simulink model "Modele_MS_V1"  (R2019b)
settings: Solver=ode23t  StartTime=0.0  StopTime=3  MaxStep=1e-3  RelTol=1e-3  EnableMultiTasking=on
InitFcn:
  | % Modelisation de la Machine Synchrone
  | 
  | % Constantes
  | 
  | Rs = 0.001;
  | Rdd = 0.01 ;
  | Rdq = Rdd ;
  | Rf = 7 ;
  | Ld = 1.59e-2 ;
  | Lq = Ld ;
  | Lf = 7 ;
  | Ldd = 7e-4 ;
  | Ldq = Ldd ;
  | Maf = 0.259 ;
  | Madd = 2.5e-3 ;
  | Madq = Madd ;
  | Mfdd = 6.8e-2 ;
  | npp = 2 ;
  | J = 0.1 ;
  | 
  | w = 2*pi*50 ;
  | 
  | Omega = w/npp ;
  | 
  | 
  | % Matrices
  | 
  | % V = [Vd Vq 0 0 Vf] ;
  | 
  | % I = [Id Iq Idd Idq If] ;
  | 
  | % F = [Fd Fq Fdd Fdq Ff] ;
  | 
  | L = [ Ld			0		Madd		0			Maf ;
  |       0			Lq		0			Madq		0 			;
  |       1.5*Madd	0		Ldd		0			Mfdd ;
  |       0        1.5*Madq			0			Ldq	0 ;
  |       1.5*Maf	0		Mfdd		0			Lf ] ;
  | 
  | L1 = inv(L) ;
  | 
  | R = [ Rs 0  0   0   0 ;
  |       0  Rs 0   0   0 ;
  |       0  0  Rdd 0   0 ;
  |       0  0  0   Rdq 0 ;
  |       0  0  0   0   Rf ] ;
  | 
  | D = [ 0 -1 0 0 0 ;
  |        1  0 0 0 0 ;
  |        0  0 0 0 0 ;
  |        0  0 0 0 0 ;
  |        0  0 0 0 0 ] ;
  | 
  |     Cl = (1/3)*[ 2  -1      -1 ;
  |      	  	        0  sqrt(3) -sqrt(3) ;
  |                   1  1       1 ] ;
  | 
  |      Cl1 = inv(Cl);
  | 
  | 
  | 
  | Clark=2/3*[	1		-1/2		-1/2
  | 	        0		sqrt(3)/2	-sqrt(3)/2
  | 	        1/2		1/2		1/2		]
  | 
  | InvClark=inv(Clark)
  | 
  | LVIDE=[Ldd   Mfdd
  |         Mfdd    Lf];
  | L2=inv(LVIDE);
  | RVIDE=[Rdd   0
  |         0    Rf];
undefined symbols (not defined in the file or in its folder): Cr, Cx, g, m, rho, Rw, S, sigbuilder_block, tau
settings Model: Creator=arzande  LastModifiedBy=jpcanesin
settings DataIOCC: LimitDataPoints=on  SaveFormat=Array  SignalLoggingSaveFormat=ModelDataLogs  ReturnWorkspaceOutputs=off
settings OptimizationCC: ExpressionDepthLimit=2147483647  InitFltsAndDblsToZero=on  LifeSpan=inf
settings DebuggingCC: UnderspecifiedInitializationDetection=Classic  MergeDetectMultiDrivingBlocksExec=none  SolverPrmCheckMsg=warning  FcnCallInpInsideContextMsg=warning  AllowSymbolicDim=off  StateNameClashWarn=warning  SFUnexpectedBacktrackingDiag=warning  SFNoUnconditionalDefaultTransitionDiag=warning  SFExecutionAtInitializationDiag=none  ArithmeticOperatorsInVariantConditions=warning
settings HardwareCC: ProdBitPerPointer=32  ProdBitPerSizeT=32  ProdBitPerPtrDiffT=32  ProdLargestAtomicFloat=None  ProdIntDivRoundTo=Undefined  ProdEndianess=Unspecified  ProdWordSize=32  ProdHWDeviceType=32-bit Generic
settings ModelReferenceCC: PropagateSignalLabelsOutOfModel=off
settings SFSimCC: SimUseLocalCustomCode=off  CustomCodeUndefinedFunction=UseInterfaceOnly
settings RTWCC: RTWUseLocalCustomCode=off
settings CodeAppCC: StateflowObjectComments=on
settings GRTTargetCC: TargetLangStandard=C89/C90 (ANSI)  GeneratePreprocessorConditionals=Disable all  CombineOutputUpdateFcns=off  GRTInterface=on
settings ConfigComp: CovMetricSettings=dw  CovHtmlReporting=on  CovSaveCumulativeToWorkspaceVar=on  CovSaveSingleToWorkspaceVar=on  CovExternalEMLEnable=off

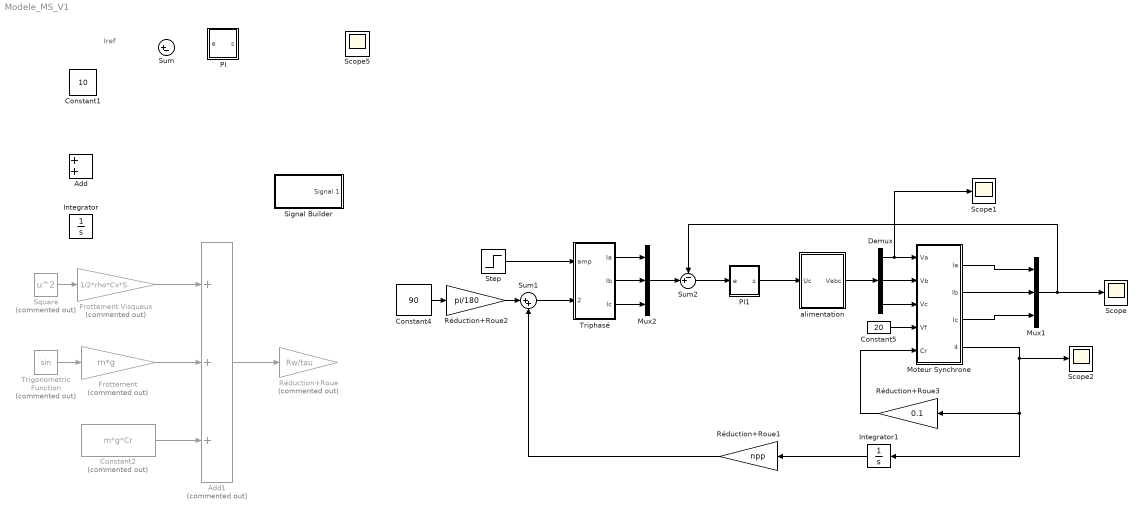
== system Modele_MS_V1 ==
  note: Iref
  Add : Sum
  Add1 : Sum  Commented=on  Inputs=+++
  Constant1 : Constant  Value=10
  Constant2 : Constant  Commented=on  Value=m*g*Cr
  Constant4 : Constant  Value=90
  Constant5 : Constant  Value=20
  Demux : Demux  Outputs=3
  "Frottement " : Gain  Commented=on  Gain=m*g
  Frottement Visqueux : Gain  Commented=on  Gain=1/2*rho*Cx*S
  Integrator : Integrator
  Integrator1 : Integrator
  Moteur Synchrone : Subsystem
  Mux1 : Mux  Inputs=3
  Mux2 : Mux  Inputs=3
  PI : Subsystem  mask{Kp=1, Ti=0.001, sat=100}
  PI1 : Subsystem  mask{Kp=1, Ti=0.001, sat=100}
  Réduction+Roue : Gain  Commented=on  Gain=Rw/tau
  Réduction+Roue1 : Gain  Gain=npp
  Réduction+Roue2 : Gain  Gain=pi/180
  Réduction+Roue3 : Gain  Gain=0.1
  Scope{,1..2,5} (4 alike) : Scope
  Signal Builder : Subsystem  Tag=STV Subsys  LoadFcn=sigbuilder_block('load');  StartFcn=sigbuilder_block('start');  StopFcn=sigbuilder_block('stop');  ClipboardFcn=sigbuilder_block('clipboard');  mask(Sigbuilder block){tuvar=[0:10]}
      mask help: Simulink:masks:SigbuilderBlock_MD
      mask init:
      | if ~strcmp(get_param(bdroot(gcbh),'SimulationStatus'),'stopped') tuvar = sigbuilder_block('maskInit'); end
      settings: CopyFcn=sigbuilder_block('copy');  DeleteFcn=sigbuilder_block('delete');  ModelCloseFcn=sigbuilder_block('modelClose');  PreSaveFcn=sigbuilder_block('preSave');  PauseFcn=sigbuilder_block('pause');  ContinueFcn=sigbuilder_block('continue');  NameChangeFcn=sigbuilder_block('namechange');  OpenFcn=sigbuilder_block('open',[406 167 550 400 ]);  CloseFcn=sigbuilder_block('close');
      mask Display: plot(0, 0, 100, 100,[2, 2, 32, 32, 2], [68, 8, 8, 68, 68],[32, 2], [38, 38], [32, 19, 2],[53, 60, 44], [32, 17, 17, 2],[16, 16, 31, 31]);txt = getActiveGroup(gcbh);text(2, 100, txt,'verticalAlignment', 'top');
  Square : Math  Commented=on  Operator=square  SignedPower=off  SaturateOnIntegerOverflow=on
  Step : Step  Time=1.2  Before=10  SampleTime=0
  Sum : Sum  Inputs=|+-  SaturateOnIntegerOverflow=on
  Sum1 : Sum  Inputs=|++  SaturateOnIntegerOverflow=on
  Sum2 : Sum  Inputs=-+|  SaturateOnIntegerOverflow=on
  Trigonometric Function : Trigonometry  Commented=on
  Triphasé : Subsystem
  alimentation : Subsystem
  wires:
  Frottement Visqueux/1 -> Add1/1
  Constant2/1 -> Add1/3
  "Frottement "/1 -> Add1/2
  Trigonometric Function/1 -> "Frottement "/1
  Square/1 -> Frottement Visqueux/1
  Add1/1 -> Réduction+Roue/1
  Moteur Synchrone/1(Ia) -> Mux1/1
  Moteur Synchrone/2(Ib) -> Mux1/2
  Moteur Synchrone/3(Ic) -> Mux1/3
  Sum1/1 -> Triphasé/2(THETA)
  Constant4/1 -> Réduction+Roue2/1
  Moteur Synchrone/4(Omega) -> Integrator1/1, Réduction+Roue3/1, Scope2/1
  Integrator1/1 -> Réduction+Roue1/1
  Réduction+Roue1/1 -> Sum1/2
  Triphasé/1(Ia) -> Mux2/1
  Triphasé/2(Ib) -> Mux2/2
  Triphasé/3(Ic) -> Mux2/3
  Sum2/1 -> PI1/1(e)
  PI1/1(s) -> alimentation/1(Uc)
  Demux/1 -> Scope1/1, Moteur Synchrone/1(Va)
  Demux/2 -> Moteur Synchrone/2(Vb)
  Demux/3 -> Moteur Synchrone/3(Vc)
  alimentation/1(Vabc) -> Demux/1
  Mux2/1 -> Sum2/2
  Mux1/1 -> Scope/1, Sum2/1
  Constant5/1 -> Moteur Synchrone/4(Vf)
  Réduction+Roue2/1 -> Sum1/1
  Step/1 -> Triphasé/1(amp)
  Réduction+Roue3/1 -> Moteur Synchrone/5(Cr)

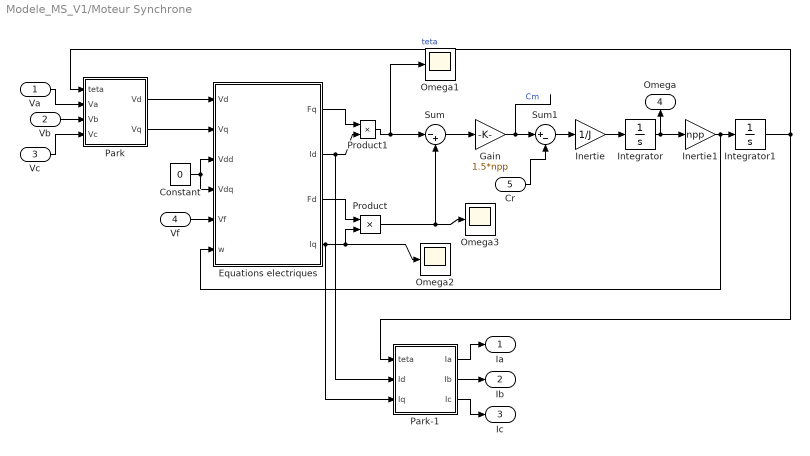
== system Modele_MS_V1/Moteur Synchrone ==
  Va : Inport
  Vb : Inport  Port=2
  Vc : Inport  Port=3
  Vf : Inport  Port=4
  Cr : Inport  Port=5
  Constant : Constant  Value=0
  Equations electriques : Subsystem
  Gain : Gain  Gain=1.5*npp  SaturateOnIntegerOverflow=on  OutDataTypeStr=Inherit: Same as input  ParamDataTypeStr=Inherit: Same as input
  Inertie : Gain  Gain=1/J  SaturateOnIntegerOverflow=on  OutDataTypeStr=Inherit: Same as input  ParamDataTypeStr=Inherit: Same as input
  Inertie1 : Gain  Gain=npp  SaturateOnIntegerOverflow=on  OutDataTypeStr=Inherit: Same as input  ParamDataTypeStr=Inherit: Same as input
  Integrator : Integrator
  Integrator1 : Integrator
  Omega1 : Scope
  Omega2 : Scope
  Omega3 : Scope
  Park : Subsystem
  Park-1 : Subsystem
  Product : Product  SaturateOnIntegerOverflow=on  InputSameDT=on  OutDataTypeStr=Inherit: Same as first input
  Product1 : Product  SaturateOnIntegerOverflow=on  InputSameDT=on  OutDataTypeStr=Inherit: Same as first input
  Sum : Sum  Inputs=|-+  SaturateOnIntegerOverflow=on  InputSameDT=on  OutDataTypeStr=Inherit: Same as first input
  Sum1 : Sum  Inputs=|+-  SaturateOnIntegerOverflow=on  InputSameDT=on  OutDataTypeStr=Inherit: Same as first input
  Ia : Outport
  Ib : Outport  Port=2
  Ic : Outport  Port=3
  Omega : Outport  Port=4
  wires:
  Equations electriques/3(Fd) -> Product/1
  Equations electriques/1(Fq) -> Product1/1
  Product/1 -> Sum/2, Omega3/1
  Product1/1 -> Sum/1, Omega1/1
  Sum/1 -> Gain/1
  Gain/1 -> Sum1/1  "Cm"
  Sum1/1 -> Inertie/1
  Inertie/1 -> Integrator/1
  Integrator/1 -> Inertie1/1, Omega/1
  Park/1(Vd) -> Equations electriques/1(Vd)
  Park/2(Vq) -> Equations electriques/2(Vq)
  Constant/1 -> Equations electriques/3(Vdd), Equations electriques/4(Vdq)
  Inertie1/1 -> Integrator1/1, Equations electriques/6(w)
  Va/1 -> Park/2(Va)
  Vb/1 -> Park/3(Vb)
  Vc/1 -> Park/4(Vc)
  Cr/1 -> Sum1/2
  Vf/1 -> Equations electriques/5(Vf)
  Park-1/1(Ia) -> Ia/1
  Park-1/2(Ib) -> Ib/1
  Park-1/3(Ic) -> Ic/1
  Equations electriques/2(Id) -> Product1/2, Park-1/2(Id)
  Equations electriques/4(Iq) -> Park-1/3(Iq), Product/2, Omega2/1
  Integrator1/1 -> Park/1(teta), Park-1/1(teta)  "teta"

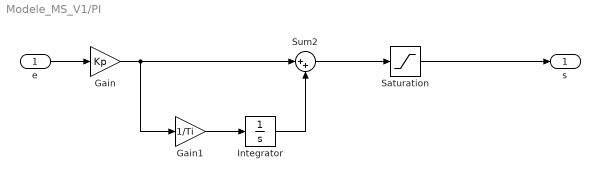
== system Modele_MS_V1/PI ==
  e : Inport
  Gain : Gain  Gain=Kp  SaturateOnIntegerOverflow=on  OutDataTypeStr=Inherit: Same as input  ParamDataTypeStr=Inherit: Same as input
  Gain1 : Gain  Gain=1/Ti  SaturateOnIntegerOverflow=on  OutDataTypeStr=Inherit: Same as input  ParamDataTypeStr=Inherit: Same as input
  Integrator : Integrator
  Saturation : Saturate  UpperLimit=sat  LowerLimit=-sat
  Sum2 : Sum  Inputs=|++  SaturateOnIntegerOverflow=on  InputSameDT=on  OutDataTypeStr=Inherit: Same as first input
  s : Outport
  wires:
  Saturation/1 -> s/1
  Sum2/1 -> Saturation/1
  Integrator/1 -> Sum2/2
  Gain1/1 -> Integrator/1
  e/1 -> Gain/1
  Gain/1 -> Gain1/1, Sum2/1

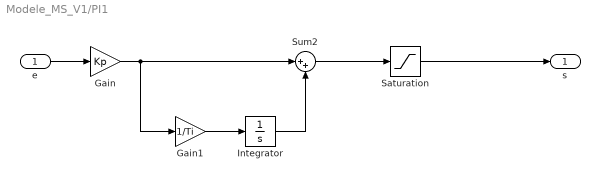
== system Modele_MS_V1/PI1 ==
  e : Inport
  Gain : Gain  Gain=Kp  SaturateOnIntegerOverflow=on  OutDataTypeStr=Inherit: Same as input  ParamDataTypeStr=Inherit: Same as input
  Gain1 : Gain  Gain=1/Ti  SaturateOnIntegerOverflow=on  OutDataTypeStr=Inherit: Same as input  ParamDataTypeStr=Inherit: Same as input
  Integrator : Integrator
  Saturation : Saturate  UpperLimit=sat  LowerLimit=-sat
  Sum2 : Sum  Inputs=|++  SaturateOnIntegerOverflow=on  InputSameDT=on  OutDataTypeStr=Inherit: Same as first input
  s : Outport
  wires:
  Saturation/1 -> s/1
  Sum2/1 -> Saturation/1
  Integrator/1 -> Sum2/2
  Gain1/1 -> Integrator/1
  e/1 -> Gain/1
  Gain/1 -> Gain1/1, Sum2/1

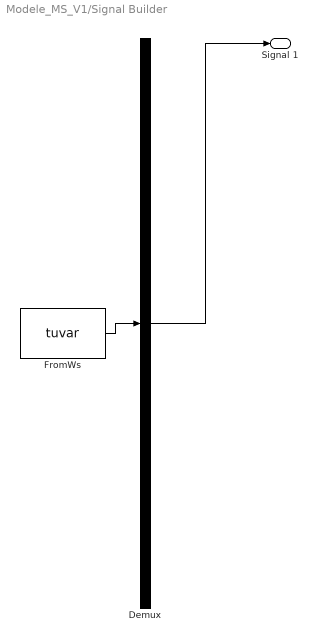
== system Modele_MS_V1/Signal Builder ==
  Demux : Demux  Tag=STV Demux  Outputs=1
  FromWs : FromWorkspace  Tag=STV FromWs  VariableName=tuvar  SampleTime=0
      SigBuilderData=|
      | common.afterFinalStr = 'Extrapolate'
      | common.sampleTime = 0
      | dataSet.timeRange = [0 10]
      | dataSet.name = 'Group 1'
      | sbobj.Groups.Name = 'Group 1'
      | sbobj.Groups.Signals.Name = 'Signal 1'
      | sbobj.Groups.Signals.XData = [0 4 4 6 6 10]
      | sbobj.Groups.Signals.YData = [0.135 0.135 1 1 0 0]
  Signal 1 : Outport  Tag=STV Outport
  wires:
  Demux/1 -> Signal 1/1
  FromWs/1 -> Demux/1

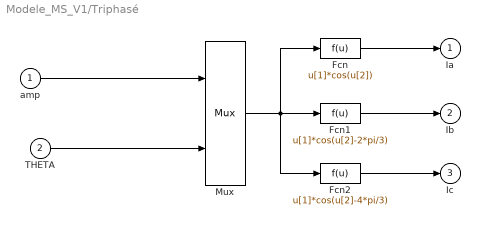
== system Modele_MS_V1/Triphasé ==
  amp : Inport
  THETA : Inport  Port=2
  Fcn : Fcn  Expr=u[1]*cos(u[2])
  Fcn1 : Fcn  Expr=u[1]*cos(u[2]-2*pi/3)
  Fcn2 : Fcn  Expr=u[1]*cos(u[2]-4*pi/3)
  Mux : Mux  Inputs=2
  Ia : Outport  InitialOutput=0
  Ib : Outport  Port=2  InitialOutput=0
  Ic : Outport  Port=3  InitialOutput=0
  wires:
  Mux/1 -> Fcn2/1, Fcn1/1, Fcn/1
  Fcn/1 -> Ia/1
  amp/1 -> Mux/1
  Fcn1/1 -> Ib/1
  Fcn2/1 -> Ic/1
  THETA/1 -> Mux/2

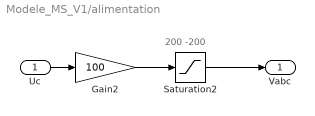
== system Modele_MS_V1/alimentation ==
  note: 200 -200
  Uc : Inport
  Gain2 : Gain  Gain=100  SaturateOnIntegerOverflow=on  OutDataTypeStr=Inherit: Same as input  ParamDataTypeStr=Inherit: Same as input
  Saturation2 : Saturate  UpperLimit=200  LowerLimit=-200
  Vabc : Outport
  wires:
  Gain2/1 -> Saturation2/1
  Uc/1 -> Gain2/1
  Saturation2/1 -> Vabc/1

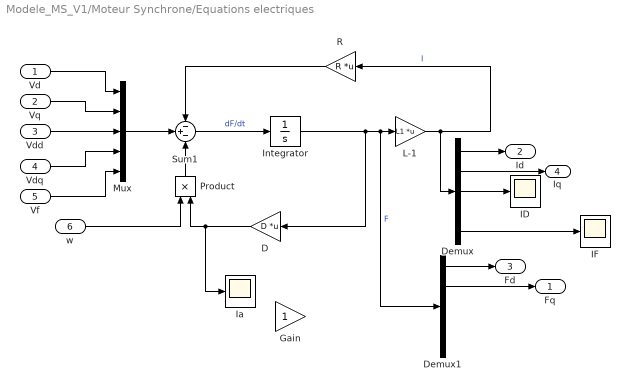
== system Modele_MS_V1/Moteur Synchrone/Equations electriques ==
  Vd : Inport
  Vq : Inport  Port=2
  Vdd : Inport  Port=3
  Vdq : Inport  Port=4
  Vf : Inport  Port=5
  w : Inport  Port=6
  D : Gain  Gain=D  Multiplication=Matrix(K*u)  SaturateOnIntegerOverflow=on  OutDataTypeStr=Inherit: Same as input  ParamDataTypeStr=Inherit: Same as input
  Demux : Demux  Outputs=5
  Demux1 : Demux  Outputs=5
  Gain : Gain
  ID : Scope
  IF : Scope
  Ia : Scope
  Integrator : Integrator
  L-1 : Gain  Gain=L1  Multiplication=Matrix(K*u)  SaturateOnIntegerOverflow=on  OutDataTypeStr=Inherit: Same as input  ParamDataTypeStr=Inherit: Same as input
  Mux : Mux  Inputs=5
  Product : Product  SaturateOnIntegerOverflow=on  InputSameDT=on  OutDataTypeStr=Inherit: Same as first input
  R : Gain  Gain=R  Multiplication=Matrix(K*u)  SaturateOnIntegerOverflow=on  OutDataTypeStr=Inherit: Same as input  ParamDataTypeStr=Inherit: Same as input
  Sum1 : Sum  Inputs=-+-  SaturateOnIntegerOverflow=on  InputSameDT=on  OutDataTypeStr=Inherit: Same as first input
  Fq : Outport
  Id : Outport  Port=2
  Fd : Outport  Port=3
  Iq : Outport  Port=4
  wires:
  Vdd/1 -> Mux/3
  Vd/1 -> Mux/1
  Vq/1 -> Mux/2
  Vdq/1 -> Mux/4
  Sum1/1 -> Integrator/1  "dF/dt"
  Mux/1 -> Sum1/2
  R/1 -> Sum1/1
  Integrator/1 -> D/1, L-1/1, Demux1/1  "F"
  L-1/1 -> R/1, Demux/1  "I"
  Vf/1 -> Mux/5
  Product/1 -> Sum1/3
  w/1 -> Product/1
  D/1 -> Product/2, Ia/1
  Demux/1 -> Id/1
  Demux/2 -> Iq/1
  Demux1/1 -> Fd/1
  Demux1/2 -> Fq/1
  Demux/5 -> IF/1
  Demux/3 -> ID/1

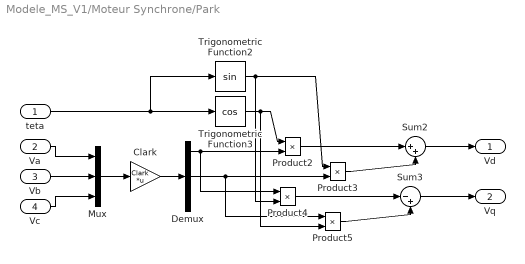
== system Modele_MS_V1/Moteur Synchrone/Park ==
  teta : Inport
  Va : Inport  Port=2
  Vb : Inport  Port=3
  Vc : Inport  Port=4
  Clark : Gain  Gain=Clark  Multiplication=Matrix(K*u)  SaturateOnIntegerOverflow=on  OutDataTypeStr=Inherit: Same as input  ParamDataTypeStr=Inherit: Same as input
  Demux : Demux  Outputs=3
  Mux : Mux  Inputs=3
  Product{2..5} (4 alike) : Product  SaturateOnIntegerOverflow=on  InputSameDT=on  OutDataTypeStr=Inherit: Same as first input
  Sum2 : Sum  Inputs=|++  SaturateOnIntegerOverflow=on  InputSameDT=on  OutDataTypeStr=Inherit: Same as first input
  Sum3 : Sum  Inputs=|-+  SaturateOnIntegerOverflow=on  InputSameDT=on  OutDataTypeStr=Inherit: Same as first input
  Trigonometric Function2 : Trigonometry
  Trigonometric Function3 : Trigonometry  Operator=cos
  Vd : Outport
  Vq : Outport  Port=2
  wires:
  Va/1 -> Mux/1
  Vb/1 -> Mux/2
  Vc/1 -> Mux/3
  Mux/1 -> Clark/1
  Clark/1 -> Demux/1
  teta/1 -> Trigonometric Function3/1, Trigonometric Function2/1
  Product2/1 -> Sum2/1
  Product3/1 -> Sum2/2
  Sum2/1 -> Vd/1
  Demux/1 -> Product2/2, Product4/1
  Trigonometric Function2/1 -> Product3/1, Product4/2
  Product4/1 -> Sum3/1
  Trigonometric Function3/1 -> Product2/1, Product5/2
  Product5/1 -> Sum3/2
  Sum3/1 -> Vq/1
  Demux/2 -> Product3/2, Product5/1

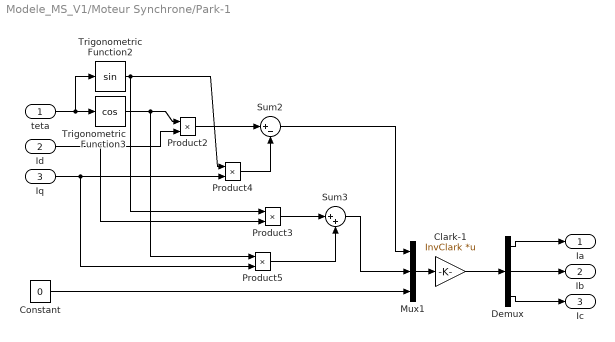
== system Modele_MS_V1/Moteur Synchrone/Park-1 ==
  teta : Inport
  Id : Inport  Port=2
  Iq : Inport  Port=3
  Clark-1 : Gain  Gain=InvClark  Multiplication=Matrix(K*u)  SaturateOnIntegerOverflow=on  OutDataTypeStr=Inherit: Same as input  ParamDataTypeStr=Inherit: Same as input
  Constant : Constant  Value=0
  Demux : Demux  Outputs=3
  Mux1 : Mux  Inputs=3
  Product{2..5} (4 alike) : Product  SaturateOnIntegerOverflow=on  InputSameDT=on  OutDataTypeStr=Inherit: Same as first input
  Sum2 : Sum  Inputs=|+-  SaturateOnIntegerOverflow=on  InputSameDT=on  OutDataTypeStr=Inherit: Same as first input
  Sum3 : Sum  Inputs=|++  SaturateOnIntegerOverflow=on  InputSameDT=on  OutDataTypeStr=Inherit: Same as first input
  Trigonometric Function2 : Trigonometry
  Trigonometric Function3 : Trigonometry  Operator=cos
  Ia : Outport
  Ib : Outport  Port=2
  Ic : Outport  Port=3
  wires:
  teta/1 -> Trigonometric Function2/1, Trigonometric Function3/1
  Product2/1 -> Sum2/1
  Product4/1 -> Sum2/2
  Constant/1 -> Mux1/3
  Mux1/1 -> Clark-1/1
  Sum2/1 -> Mux1/1
  Id/1 -> Product2/2, Product3/2
  Trigonometric Function2/1 -> Product4/1, Product3/1
  Sum3/1 -> Mux1/2
  Product3/1 -> Sum3/1
  Trigonometric Function3/1 -> Product2/1, Product5/1
  Iq/1 -> Product4/2, Product5/2
  Product5/1 -> Sum3/2
  Clark-1/1 -> Demux/1
  Demux/1 -> Ia/1
  Demux/2 -> Ib/1
  Demux/3 -> Ic/1
